simulink model "Test"  (R2018b)
settings: Solver=FixedStepAuto  StartTime=0.0  StopTime=50  FixedStep=0.01  RelTol=1e-3
libraries: simulink x2
settings Model: Creator=DwigHT  LastModifiedBy=DwigHT

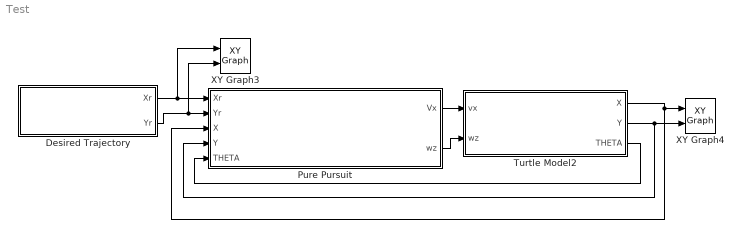
== system Test ==
  Desired Trajectory : Subsystem
  Pure Pursuit : Subsystem
  Turtle Model2 : Subsystem
  XY Graph3 : simulink/Sinks/XY Graph  xmin=0  xmax=11  ymin=0  ymax=11  st=-1
  XY Graph4 : simulink/Sinks/XY Graph  xmin=0  xmax=11  ymin=0  ymax=11  st=-1
  wires:
  Turtle Model2/2(Y) -> Pure Pursuit/4(Y), XY Graph4/2
  Pure Pursuit/2(wz) -> Turtle Model2/2(wz)
  Turtle Model2/1(X) -> Pure Pursuit/3(X), XY Graph4/1
  Turtle Model2/3(THETA) -> Pure Pursuit/5(THETA)
  Desired Trajectory/1(Xr) -> Pure Pursuit/1(Xr), XY Graph3/1
  Pure Pursuit/1(Vx) -> Turtle Model2/1(vx)
  Desired Trajectory/2(Yr) -> Pure Pursuit/2(Yr), XY Graph3/2

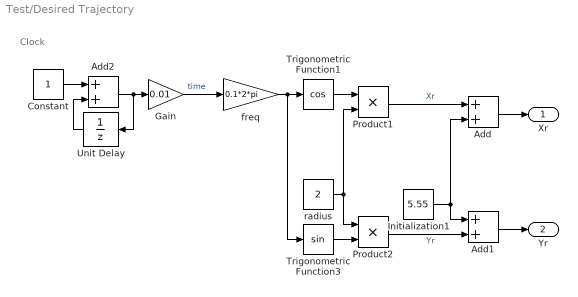
== system Test/Desired Trajectory ==
  note: Clock
  Add : Sum
  Add1 : Sum
  Add2 : Sum
  Constant : Constant
  Gain : Gain  Gain=0.01
  Initialization1 : Constant  Value=5.55
  Product1 : Product  RndMeth=Zero
  Product2 : Product  RndMeth=Zero
  Trigonometric Function1 : Trigonometry  Operator=cos
  Trigonometric Function3 : Trigonometry
  Unit Delay : UnitDelay  SampleTime=0.01
  freq : Gain  Gain=0.1*2*pi
  radius : Constant  Value=2
  Xr : Outport
  Yr : Outport  Port=2
  wires:
  Initialization1/1 -> Add/2, Add1/1
  radius/1 -> Product2/1, Product1/2
  Add1/1 -> Yr/1
  freq/1 -> Trigonometric Function3/1, Trigonometric Function1/1
  Trigonometric Function3/1 -> Product2/2
  Trigonometric Function1/1 -> Product1/1
  Product1/1 -> Add/1  "Xr"
  Product2/1 -> Add1/2  "Yr"
  Add/1 -> Xr/1
  Gain/1 -> freq/1  "time"
  Add2/1 -> Unit Delay/1, Gain/1
  Unit Delay/1 -> Add2/2
  Constant/1 -> Add2/1

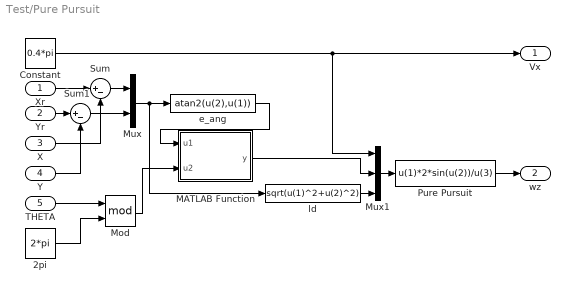
== system Test/Pure Pursuit ==
  Xr : Inport
  Yr : Inport  Port=2
  X : Inport  Port=3
  Y : Inport  Port=4
  THETA : Inport  Port=5
  2pi : Constant  Value=2*pi
  Constant : Constant  Value=0.4*pi
  MATLAB Function : MATLAB Function  TreatAsAtomicUnit=on
  Mod : Math  Operator=mod  SaturateOnIntegerOverflow=on
  Mux : Mux  Inputs=2
  Mux1 : Mux  Inputs=3
  Pure Pursuit : Fcn  Expr=u(1)*2*sin(u(2))/u(3)
  Sum : Sum  Inputs=|+-
  Sum1 : Sum  Inputs=|+-
  e_ang : Fcn  Expr=atan2(u(2),u(1))
  ld : Fcn  Expr=sqrt(u(1)^2+u(2)^2)
  Vx : Outport
  wz : Outport  Port=2
  wires:
  THETA/1 -> Mod/1
  X/1 -> Sum/2
  Xr/1 -> Sum/1
  Yr/1 -> Sum1/1
  Mux/1 -> e_ang/1, ld/1
  Pure Pursuit/1 -> wz/1
  ld/1 -> Mux1/3
  MATLAB Function/1(y) -> Mux1/2
  Sum/1 -> Mux/1
  e_ang/1 -> MATLAB Function/1(u1)
  Y/1 -> Sum1/2
  Mux1/1 -> Pure Pursuit/1
  Sum1/1 -> Mux/2
  Constant/1 -> Vx/1, Mux1/1
  Mod/1 -> MATLAB Function/2(u2)
  2pi/1 -> Mod/2

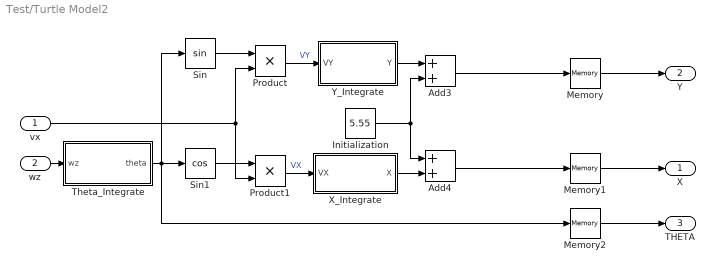
== system Test/Turtle Model2 ==
  vx : Inport
  wz : Inport  Port=2
  Add3 : Sum
  Add4 : Sum
  Initialization : Constant  Value=5.55
  Memory : Memory  InitialCondition=5.55  InheritSampleTime=on
  Memory1 : Memory  InitialCondition=5.55  InheritSampleTime=on
  Memory2 : Memory  InheritSampleTime=on
  Product : Product
  Product1 : Product
  Sin : Trigonometry
  Sin1 : Trigonometry  Operator=cos
  Theta_Integrate : Subsystem
  X_Integrate : Subsystem
  Y_Integrate : Subsystem
  X : Outport
  Y : Outport  Port=2
  THETA : Outport  Port=3
  wires:
  Memory2/1 -> THETA/1
  Memory1/1 -> X/1
  Memory/1 -> Y/1
  vx/1 -> Product/2, Product1/2
  Initialization/1 -> Add4/1, Add3/2
  Sin/1 -> Product/1
  Sin1/1 -> Product1/1
  Add4/1 -> Memory1/1
  Theta_Integrate/1(theta) -> Sin/1, Memory2/1, Sin1/1
  wz/1 -> Theta_Integrate/1(wz)
  Product/1 -> Y_Integrate/1(VY)  "VY"
  Y_Integrate/1(Y) -> Add3/1
  Product1/1 -> X_Integrate/1(VX)  "VX"
  X_Integrate/1(X) -> Add4/2
  Add3/1 -> Memory/1

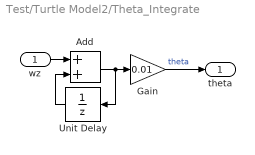
== system Test/Turtle Model2/Theta_Integrate ==
  wz : Inport
  Add : Sum
  Gain : Gain  Gain=0.01
  Unit Delay : UnitDelay  SampleTime=0.01
  theta : Outport
  wires:
  Gain/1 -> theta/1  "theta"
  Add/1 -> Gain/1, Unit Delay/1
  Unit Delay/1 -> Add/2
  wz/1 -> Add/1

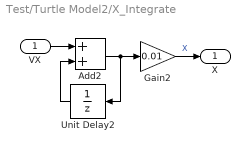
== system Test/Turtle Model2/X_Integrate ==
  VX : Inport
  Add2 : Sum
  Gain2 : Gain  Gain=0.01
  Unit Delay2 : UnitDelay  SampleTime=0.01
  X : Outport
  wires:
  Unit Delay2/1 -> Add2/2
  Add2/1 -> Gain2/1, Unit Delay2/1
  Gain2/1 -> X/1  "X"
  VX/1 -> Add2/1

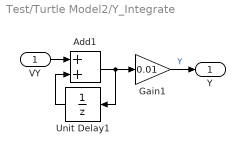
== system Test/Turtle Model2/Y_Integrate ==
  VY : Inport
  Add1 : Sum
  Gain1 : Gain  Gain=0.01
  Unit Delay1 : UnitDelay  SampleTime=0.01
  Y : Outport
  wires:
  Gain1/1 -> Y/1  "Y"
  Unit Delay1/1 -> Add1/2
  Add1/1 -> Gain1/1, Unit Delay1/1
  VY/1 -> Add1/1

== matlab function Test/Pure Pursuit/MATLAB Function ==
  data: u1 input; y output; u2 input
function y = fcn(u1,u2)
if u1<0
    u1=2*pi+u1;
end
y = u1-u2;
